simulink model "Hypotenuse_solution"  (R2018a)
settings: Solver=VariableStepAuto  StartTime=0.0  StopTime=10.0  RelTol=1e-3
settings Model: Creator=josea  LastModifiedBy=josea

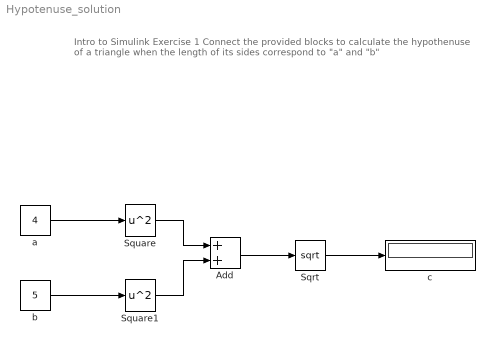
== system Hypotenuse_solution ==
  note: Intro to Simulink Exercise 1
      |
      | Connect the provided blocks to calculate the hypothenuse of a triangle when the length of its sides correspond to "a" and "b"
  Add : Sum
  Sqrt : Sqrt  SaturateOnIntegerOverflow=on
  Square : Math  Operator=square  SaturateOnIntegerOverflow=on
  Square1 : Math  Operator=square  SaturateOnIntegerOverflow=on
  a : Constant  Value=4
  b : Constant  Value=5
  c : Display
  wires:
  a/1 -> Square/1
  b/1 -> Square1/1
  Square/1 -> Add/1
  Square1/1 -> Add/2
  Add/1 -> Sqrt/1
  Sqrt/1 -> c/1
